simulink library "calcTangentRollAngle_ul"  (R2020a)
settings: Solver=VariableStepAuto  StartTime=0.0  StopTime=10.0  RelTol=1e-3
settings Model: Creator=Ayaz  LastModifiedBy=Ayaz

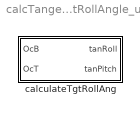
== system calcTangentRollAngle_ul ==
  calculateTgtRollAng : Subsystem

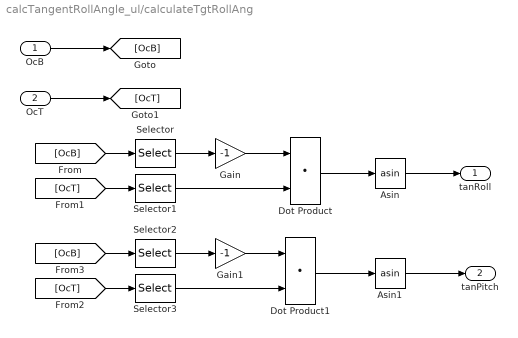
== system calcTangentRollAngle_ul/calculateTgtRollAng ==
  OcB : Inport
  OcT : Inport  Port=2
  Asin : Trigonometry  Operator=asin
  Asin1 : Trigonometry  Operator=asin
  Dot Product : DotProduct  InputSameDT=on  OutDataTypeStr=Inherit: Inherit via internal rule
  Dot Product1 : DotProduct  InputSameDT=on  OutDataTypeStr=Inherit: Inherit via internal rule
  Gain : Gain  Gain=-1
  Gain1 : Gain  Gain=-1
  Selector : Selector  NumberOfDimensions=2  InputPortWidth=3  IndexOptions=Index vector (dialog),Index vector (dialog)  Indices=[1 2 3],2  OutputSizes=1,1
  Selector1 : Selector  NumberOfDimensions=2  InputPortWidth=3  IndexOptions=Index vector (dialog),Index vector (dialog)  Indices=[1 2 3],3  OutputSizes=1,1
  Selector2 : Selector  NumberOfDimensions=2  InputPortWidth=3  IndexOptions=Index vector (dialog),Index vector (dialog)  Indices=[1 2 3],1  OutputSizes=1,1
  Selector3 : Selector  NumberOfDimensions=2  InputPortWidth=3  IndexOptions=Index vector (dialog),Index vector (dialog)  Indices=[1 2 3],3  OutputSizes=1,1
  tanRoll : Outport
  tanPitch : Outport  Port=2
  wires:
  OcT/1 -> [OcT]
  Selector/1 -> Gain/1
  Selector1/1 -> Dot Product/2
  Asin/1 -> tanRoll/1
  Gain/1 -> Dot Product/1
  Dot Product/1 -> Asin/1
  OcB/1 -> [OcB]
  [OcB] -> Selector/1
  [OcT] -> Selector1/1
  [OcB] -> Selector2/1
  Selector2/1 -> Gain1/1
  Gain1/1 -> Dot Product1/1
  [OcT] -> Selector3/1
  Selector3/1 -> Dot Product1/2
  Dot Product1/1 -> Asin1/1
  Asin1/1 -> tanPitch/1
